simulink model "Rigid_Body_Spacecraft"  (R2021b)
settings: Solver=VariableStepAuto  StartTime=0.0  StopTime=10  RelTol=1e-3
values from neighbouring files (symbols this model uses):
  Gd = 0.9    [Experiment_5.m]
  Gp = 1    [Experiment_5.m]
  I = 0.1    [Experiment_5.m]
settings Model: Creator=William Watkins  LastModifiedBy=William Watkins

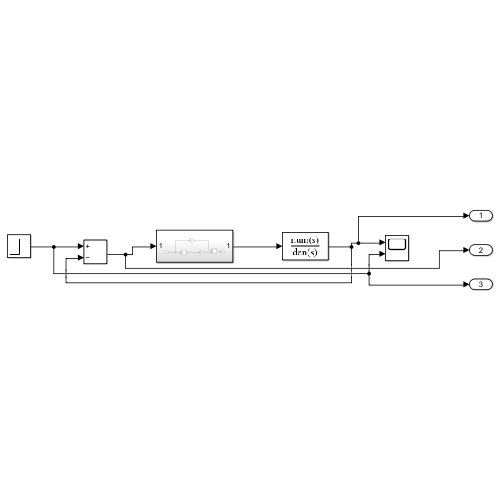
[thumbnail: Simulink's stored preview of the top-level diagram]
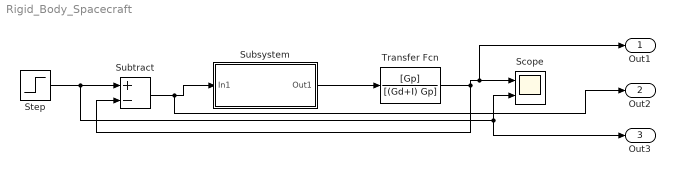
== system Rigid_Body_Spacecraft ==
  Scope : Scope  NumInputPorts=2
  Step : Step  After=0.4  SampleTime=0
  Subsystem : Subsystem
  Subtract : Sum  Inputs=+-
  Transfer Fcn : TransferFcn  Numerator=[Gp]  Denominator=[(Gd+I) Gp]
  Out1 : Outport
  Out2 : Outport  Port=2
  Out3 : Outport  Port=3
  wires:
  Step/1 -> Scope/2, Out3/1, Subtract/1
  Subsystem/1(Out1) -> Transfer Fcn/1
  Transfer Fcn/1 -> Out1/1, Scope/1, Subtract/2
  Subtract/1 -> Out2/1, Subsystem/1(In1)

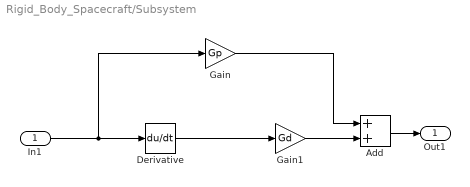
== system Rigid_Body_Spacecraft/Subsystem ==
  In1 : Inport
  Add : Sum
  Derivative : Derivative
  Gain : Gain  Gain=Gp
  Gain1 : Gain  Gain=Gd
  Out1 : Outport
  wires:
  In1/1 -> Gain/1, Derivative/1
  Derivative/1 -> Gain1/1
  Gain1/1 -> Add/2
  Add/1 -> Out1/1
  Gain/1 -> Add/1
